simulink model "Golf_Nonlin_ClassiqueDEMO"  (R2019a)
settings: Solver=VariableStepAuto  StartTime=0.0  StopTime=7  RelTol=1e-3
values from neighbouring files (symbols this model uses):
  DEG2RAD = pi/180.    (= 0.0174532925199)    [mainProjetCADV_2a.m]    (also in utAcDynamicsFunction.m; utConstantAeroCoeff.m)
  dPHRTrim = trimVal(1)    [mainProjetCADV_2a.m]
  dthrIdle = 0.1    [mainProjetCADV_2a.m]
  km = trim.kmass(choix)    [utGetTrimPoint.m]
  ms = trim.mStat(choix)    [utGetTrimPoint.m]
  RAD2DEG = 180/pi    (= 57.2957795131)    [mainProjetCADV_2a.m]    (also in utAcDynamicsFunction.m)
  thetaTrim = trimVal(3)    [mainProjetCADV_2a.m]
  uTrim = zeros(TOTAL_CMD, 1)    [mainProjetCADV_2a.m]
  xTrim = zeros(TOTAL_SV, 1)    [mainProjetCADV_2a.m]
undefined symbols (not defined in the file or in its folder): aircraftChosen, Cpf, Kd, Ki, Kp, state4den, state4num
libraries: simulink x1
settings Model: Creator=bourdiul  LastModifiedBy=ulyss

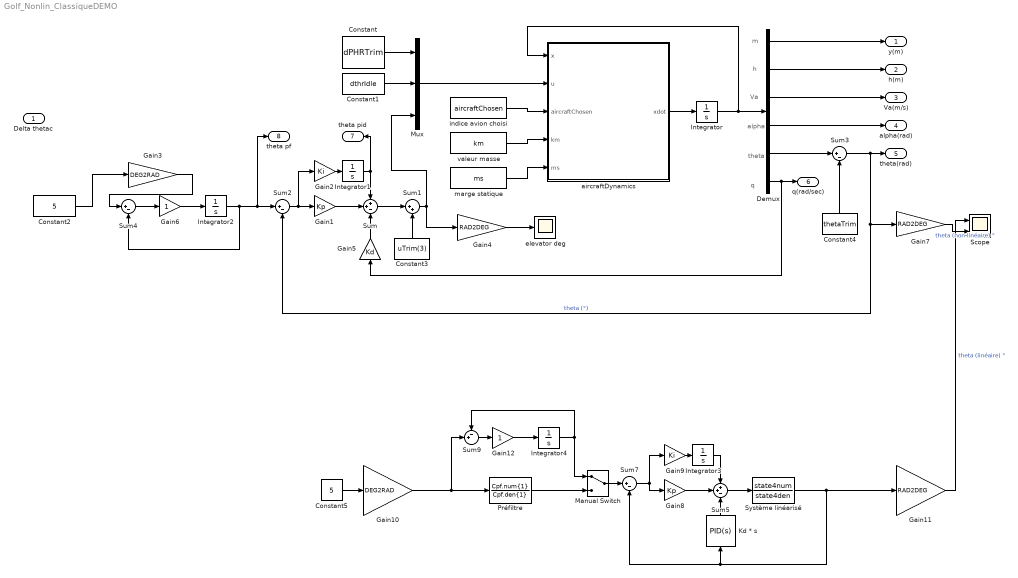
== system Golf_Nonlin_ClassiqueDEMO ==
  note: m
  note: h
  note: Va
  note: alpha
  note: theta
  note: q
  "Delta thetac " : Inport
  Constant : Constant  Value=dPHRTrim
  Constant1 : Constant  Value=dthrIdle
  Constant2 : Constant  Value=5
  Constant3 : Constant  Value=uTrim(3)
  Constant4 : Constant  Value=thetaTrim
  Constant5 : Constant  Value=5
  Demux : Demux  Outputs=6
  Gain1 : Gain  Gain=Kp
  Gain10 : Gain  Gain=DEG2RAD
  Gain11 : Gain  Gain=RAD2DEG
  Gain12 : Gain
  Gain2 : Gain  Gain=Ki
  Gain3 : Gain  Gain=DEG2RAD
  Gain4 : Gain  Gain=RAD2DEG
  Gain5 : Gain  Gain=Kd
  Gain6 : Gain
  Gain7 : Gain  Gain=RAD2DEG
  Gain8 : Gain  Gain=Kp
  Gain9 : Gain  Gain=Ki
  Integrator : Integrator  InitialCondition=xTrim
  Integrator{1..4} (4 alike) : Integrator
  Kd * s : simulink/Continuous/PID Controller  Controller=PID  Form=Parallel  TimeDomain=Continuous-time  SampleTime=-1  IntegratorMethod=Forward Euler  FilterMethod=Forward Euler  ControllerParametersSource=internal  P=0  I=0  D=Kd  UseFilter=on  N=100  TunerSelectOption=Transfer Function Based (PID Tuner App)  InitialConditionSource=internal  InitialConditionForIntegrator=0  InitialConditionForFilter=0  DifferentiatorICPrevScaledInput=0  ExternalReset=none  TrackingMode=off  Kt=1  LimitOutput=off  UpperSaturationLimit=inf  LowerSaturationLimit=-inf  LinearizeAsGain=on  AntiWindupMode=none  Kb=1  POutMin=[]  POutMax=[]  IOutMin=[]  IOutMax=[]  DOutMin=[]  DOutMax=[]  NOutMin=[]  NOutMax=[]  SumOutMin=[]  SumOutMax=[]  SaturationOutMin=[]  SaturationOutMax=[]  PParamMin=[]  PParamMax=[]  IParamMin=[]  IParamMax=[]  DParamMin=[]  DParamMax=[]  NParamMin=[]  NParamMax=[]  KbParamMin=[]  KbParamMax=[]  KtParamMin=[]  KtParamMax=[]  KbOutMin=[]  KbOutMax=[]  KtOutMin=[]  KtOutMax=[]  IntegratorOutMin=[]  IntegratorOutMax=[]  FilterOutMin=[]  FilterOutMax=[]  SumI1OutMin=[]  SumI1OutMax=[]  SumI2OutMin=[]  SumI2OutMax=[]  SumI3OutMin=[]  SumI3OutMax=[]  SumI4OutMin=[]  SumI4OutMax=[]  SumDOutMin=[]  SumDOutMax=[]  DifferentiatorOutMin=[]  DifferentiatorOutMax=[]  FilterDiffOutCoefMin=[]  FilterDiffOutCoefMax=[]  ReciprocalOutMin=[]  ReciprocalOutMax=[]  SumDenOutMin=[]  SumDenOutMax=[]  SumNumOutMin=[]  SumNumOutMax=[]  DivideOutMin=[]  DivideOutMax=[]  IntegratorContinuousStateAttributes=''  IntegratorStateMustResolveToSignalObject=off  IntegratorRTWStateStorageClass=Auto  FilterContinuousStateAttributes=''  FilterStateMustResolveToSignalObject=off  FilterRTWStateStorageClass=Auto  ParallelPVariant=InternalParameters  IdealPVariant=Disabled  IVariant=InternalParameters  DVariant=InternalParameters  IntegratorVariant=Continuous  SatVariant=Disabled  AWVariant=Passthrough  PCopyVariant=Disabled  TRVariant=Disabled  FdbkBlocksVariant=Forward  IdealPFdbkVariant=Disabled  SatFdbkVariant=Disabled  DerivativeFilterVariant=ContFilter  NVariant=InternalParameters  NCopyVariant=Disabled  FilterICVariant=InternalICsFilter  IntegratorICVariant=InternalICs  ExternalResetVariant=Disabled  TRSumVariant=Passthrough  SumFdbkVariant=Disabled  SumVariant=Sum_PID
  Manual Switch : ManualSwitch
  Mux : Mux  Inputs=3
  Préfiltre : TransferFcn  Numerator=Cpf.num{1}  Denominator=Cpf.den{1}
  Scope : Scope  NumInputPorts=2
  Sum : Sum  Inputs=++-
  Sum1 : Sum  Inputs=|++
  Sum{2..4,7} (4 alike) : Sum  Inputs=|+-
  Sum5 : Sum  Inputs=++-
  Sum9 : Sum  Inputs=-+|
  Système linéarisé : TransferFcn  Numerator=state4num  Denominator=state4den
  aircraftDynamics : MATLAB Function  TreatAsAtomicUnit=on
  elevator deg : Scope
  indice avion choisi : Constant  Value=aircraftChosen
  marge statique : Constant  Value=ms
  valeur masse : Constant  Value=km
  y(m) : Outport
  h(m) : Outport  Port=2
  Va(m/s) : Outport  Port=3
  alpha(rad) : Outport  Port=4
  theta(rad) : Outport  Port=5
  q(rad/sec) : Outport  Port=6
  theta pid : Outport  Port=7
  "theta pf " : Outport  Port=8
  wires:
  marge statique/1 -> aircraftDynamics/5(ms)
  Integrator/1 -> Demux/1, aircraftDynamics/1(x)
  Demux/6 -> Gain5/1, q(rad/sec)/1
  Mux/1 -> aircraftDynamics/2(u)
  Demux/2 -> h(m)/1
  indice avion choisi/1 -> aircraftDynamics/3(aircraftChosen)
  Demux/3 -> Va(m/s)/1
  valeur masse/1 -> aircraftDynamics/4(km)
  aircraftDynamics/1(xdot) -> Integrator/1
  Demux/4 -> alpha(rad)/1
  Constant1/1 -> Mux/2
  Constant/1 -> Mux/1
  Demux/1 -> y(m)/1
  Gain5/1 -> Sum/3
  Gain4/1 -> elevator deg/1
  Constant4/1 -> Sum3/2
  Gain1/1 -> Sum/2
  Integrator1/1 -> theta pid/1, Sum/1
  Gain2/1 -> Integrator1/1
  Sum2/1 -> Gain2/1, Gain1/1
  Demux/5 -> Sum3/1
  Sum3/1 -> theta(rad)/1, Sum2/2, Gain7/1  "theta (°)"
  Integrator2/1 -> "theta pf "/1, Sum2/1, Sum4/2
  Gain6/1 -> Integrator2/1
  Sum4/1 -> Gain6/1
  Constant3/1 -> Sum1/2
  Sum/1 -> Sum1/1
  Sum1/1 -> Gain4/1, Mux/3
  Gain3/1 -> Sum4/1
  Gain7/1 -> Scope/2  "theta (non-linéaire) °"
  Constant2/1 -> Gain3/1
  Système linéarisé/1 -> Gain11/1, Sum7/2, Kd * s/1
  Constant5/1 -> Gain10/1
  Gain11/1 -> Scope/1  "theta (linéaire) °"
  Manual Switch/1 -> Sum7/1
  Integrator4/1 -> Manual Switch/1, Sum9/1
  Gain9/1 -> Integrator3/1
  Sum9/1 -> Gain12/1
  Sum7/1 -> Gain8/1, Gain9/1
  Gain8/1 -> Sum5/2
  Integrator3/1 -> Sum5/1
  Préfiltre/1 -> Manual Switch/2
  Gain12/1 -> Integrator4/1
  Gain10/1 -> Sum9/2, Préfiltre/1
  Kd * s/1 -> Sum5/3
  Sum5/1 -> Système linéarisé/1

== matlab function Golf_Nonlin_ClassiqueDEMO/aircraftDynamics ==
  data: x input; u input; xdot output; aircraftChosen input; km input; ms input
function xdot = aircraftDynamics(x,u, aircraftChosen,km,ms)
    TOTAL_SV = 6;
    xIn = zeros(TOTAL_SV,1);
    xIn = x;
    
	TOTAL_CMD = 3;
    uIn = zeros(TOTAL_CMD,1);
    uIn = u;
    
    xdot = utAcDynamicsFunction(xIn,uIn, aircraftChosen,km,ms);
end %aircraftDynamics
